simulink model "A2_2_Inverses_Pendel_lin"  (R2023b)
settings: Solver=FixedStepAuto  StartTime=0.0  StopTime=Te  FixedStep=Ts  RelTol=1e-3
values from neighbouring files (symbols this model uses):
  A = [0 0 1 0; 0 0 0 1; 0 0.1e1 / CM / ig ^ 2 * c 0 0; 0 -(CM * ig ^ 2 + ms * s ^ 2 + CA) / CM / ig ^ 2 / (ms * s ^ 2 + CA) * c 0 0;]    [init_DSMS.m]    (also in init_DSMS_vorlage.m = [ 0 1 ; -c/m -d/m ]; init_elast_Getriebe.m = [0 0 1 0; 0 0 0 1; 0 0.1e1 / C_M_S / ig ^ 2 * c -0.1e1 / C_M; init_inverse_pendel_lin.m = [0 0 1 0; 0 0 0 1; 0 12 * m2 * s2 ^ 2 * g * l1 / (12 * (C_M_; init_inverse_pendel_pr.m = [0 0 0 1 0 0; 0 0 0 0 1 0; 0 0 0 0 0 1; 0 0.12e2 * l1 * g * )
  B = [0; 0; 0.1e1 / CM / ig; -0.1e1 / CM / ig;]    [init_DSMS.m]    (also in init_DSMS_vorlage.m = [ 0 1/m ]'; init_elast_Getriebe.m = [0; 0; 0.1e1 / C_M_S / ig; -0.1e1 / C_M_S / ig;]; init_inverse_pendel_lin.m = [0; 0; ig * (l2 ^ 2 + 12 * s2 ^ 2) / (12 * (C_M_S * ig ^ 2 +; init_inverse_pendel_pr.m = [0 0 0; 0 0 0; 0 0 0; 0.12e2 * ig * (((mP2 * l3 ^ 2 + m3 * s)
  C = diag([1, 1, 1, 1])    [init_DSMS.m]    (also in init_DSMS_vorlage.m = diag([1, 1]); init_elast_Getriebe.m = eye(4); init_inverse_pendel_lin.m = [0, 1,0,0]; init_inverse_pendel_pr.m = eye(6))
  D = zeros(size(C,1),size(B,2))    [init_DSMS.m]    (also in init_DSMS_vorlage.m; init_elast_Getriebe.m = [0; 0; 0; 0]; init_inverse_pendel_lin.m = 0; init_inverse_pendel_pr.m = [0 0 0; 0 0 0; 0 0 0; 0 0 0; 0 0 0; 0 0 0])
  x1_ic = zeros(4,1)    [init_DSMS.m]    (also in init_DSMS_vorlage.m = zeros(2,1); init_elast_Getriebe.m; init_inv.m; init_inverse_pendel.m)
settings Model: Creator=Flo  LastModifiedBy=Flo

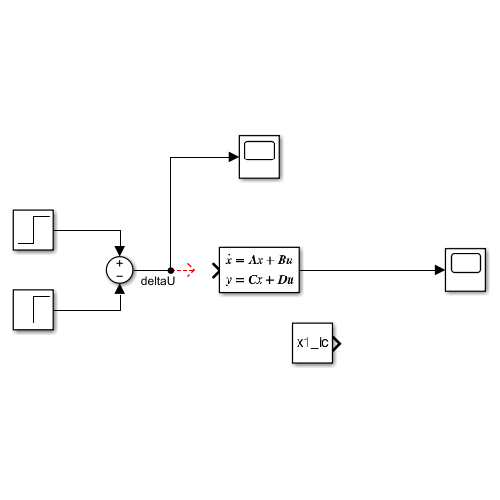
[thumbnail: Simulink's stored preview of the top-level diagram]
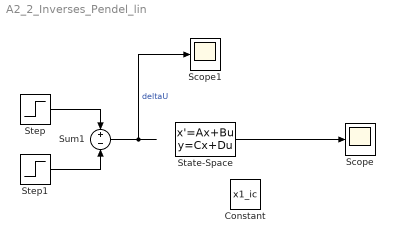
== system A2_2_Inverses_Pendel_lin ==
  Constant : Constant  Value=x1_ic
  Scope : Scope
  Scope1 : Scope
  State-Space : StateSpace  A=A  B=B  C=C  D=D  InitialCondition=[0,1,0,0]
  Step : Step  SampleTime=0
  Step1 : Step  Time=2  SampleTime=0
  Sum1 : Sum  Inputs=+-
  wires:
  State-Space/1 -> Scope/1
  Step/1 -> Sum1/1
  Step1/1 -> Sum1/2
  Sum1/1 -> Scope1/1  "deltaU"
